simulink library "variableFlowProfileCalculationYZ_ul"  (R2018b)
settings: Solver=VariableStepAuto  StartTime=0.0  StopTime=10.0  RelTol=1e-3
libraries: Dynamic_2D_Lookup_Table x3, dspmtrx3 x3
settings Model: Creator=James Reed  LastModifiedBy=jcreed2

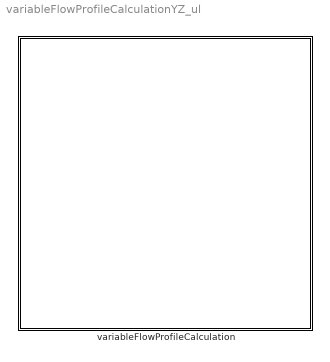
== system variableFlowProfileCalculationYZ_ul ==
  variableFlowProfileCalculation : Subsystem

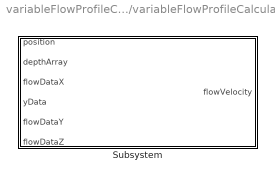
== system variableFlowProfileCalculationYZ_ul/variableFlowProfileCalculation ==
  Subsystem : Subsystem

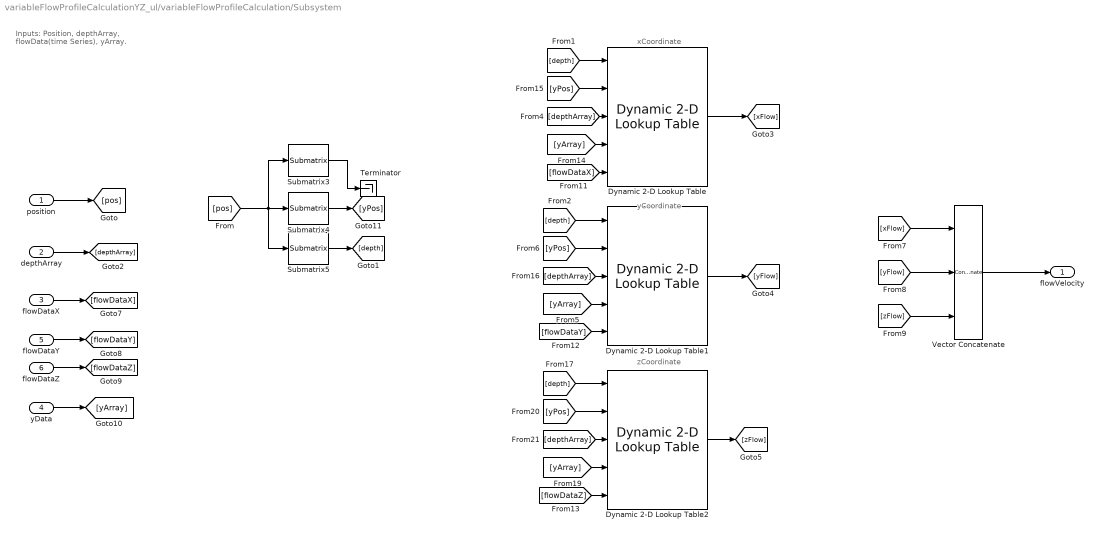
== system variableFlowProfileCalculationYZ_ul/variableFlowProfileCalculation/Subsystem ==
  note: Inputs: Position, depthArray,
      | flowData(time Series), yArray.
  note: xCoordinate
  note: zCoordinate
  note: yCoordinate
  "position " : Inport
  "depthArray " : Inport  Port=2
  "flowDataX " : Inport  Port=3
  "yData " : Inport  Port=4
  "flowDataY " : Inport  Port=5
  flowDataZ : Inport  Port=6
  Dynamic 2-D Lookup Table : Dynamic_2D_Lookup_Table/Dynamic 2-D Lookup Table
  Dynamic 2-D Lookup Table1 : Dynamic_2D_Lookup_Table/Dynamic 2-D Lookup Table
  Dynamic 2-D Lookup Table2 : Dynamic_2D_Lookup_Table/Dynamic 2-D Lookup Table
  Submatrix3 : dspmtrx3/Submatrix  RowSpan=One row  RowStartMode=First  RowStartIndex=1  RowEndMode=Last  RowEndIndex=1  ColSpan=All columns  ColStartMode=First  ColStartIndex=1  ColEndMode=Last  ColEndIndex=1
  Submatrix4 : dspmtrx3/Submatrix  RowSpan=One row  RowStartMode=First  RowStartIndex=1  RowEndMode=Last  RowEndIndex=1  ColSpan=All columns  ColStartMode=First  ColStartIndex=1  ColEndMode=Last  ColEndIndex=1
  Submatrix5 : dspmtrx3/Submatrix  RowSpan=One row  RowStartMode=First  RowStartIndex=1  RowEndMode=Last  RowEndIndex=1  ColSpan=All columns  ColStartMode=First  ColStartIndex=1  ColEndMode=Last  ColEndIndex=1
  Terminator : Terminator
  Vector Concatenate : Concatenate  NumInputs=3  Mode=Multidimensional array
  "flowVelocity " : Outport
  wires:
  Dynamic 2-D Lookup Table2/1 -> [zFlow]
  [yArray] -> Dynamic 2-D Lookup Table/4
  Dynamic 2-D Lookup Table1/1 -> [yFlow]
  [depth] -> Dynamic 2-D Lookup Table1/1
  [yPos] -> Dynamic 2-D Lookup Table1/2
  [xFlow] -> Vector Concatenate/1
  Dynamic 2-D Lookup Table/1 -> [xFlow]
  Submatrix3/1 -> Terminator/1
  [flowDataY] -> Dynamic 2-D Lookup Table1/5
  Vector Concatenate/1 -> "flowVelocity "/1
  [zFlow] -> Vector Concatenate/3
  [pos] -> Submatrix3/1, Submatrix5/1, Submatrix4/1
  [depth] -> Dynamic 2-D Lookup Table/1
  [depthArray] -> Dynamic 2-D Lookup Table2/3
  [depth] -> Dynamic 2-D Lookup Table2/1
  [flowDataZ] -> Dynamic 2-D Lookup Table2/5
  "yData "/1 -> [yArray]
  [yArray] -> Dynamic 2-D Lookup Table2/4
  [depthArray] -> Dynamic 2-D Lookup Table1/3
  [yArray] -> Dynamic 2-D Lookup Table1/4
  [yPos] -> Dynamic 2-D Lookup Table2/2
  "flowDataX "/1 -> [flowDataX]
  "position "/1 -> [pos]
  Submatrix4/1 -> [yPos]
  [yPos] -> Dynamic 2-D Lookup Table/2
  "depthArray "/1 -> [depthArray]
  [depthArray] -> Dynamic 2-D Lookup Table/3
  Submatrix5/1 -> [depth]
  [yFlow] -> Vector Concatenate/2
  [flowDataX] -> Dynamic 2-D Lookup Table/5
  "flowDataY "/1 -> [flowDataY]
  flowDataZ/1 -> [flowDataZ]
